simulink model "untitled"  (R2015b)
settings: Solver=VariableStepAuto  StartTime=0.0  StopTime=10.0  RelTol=1e-3
libraries: fl_lib x5, simulink_extras x2, simrfV2junction1 x2, commsynccomp2 x1
settings Model: Creator=dimple  LastModifiedBy=dimple

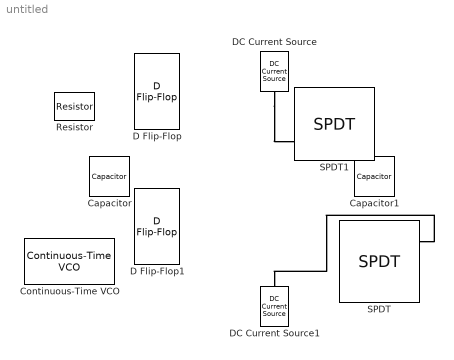
== system untitled ==
  Capacitor : fl_lib/Electrical/Electrical Elements/Capacitor  c=1e-6 F  r=1e-6 Ohm  g=0 1/Ohm  i_specify=off  i_priority=None  i=0 A  v_specify=off  v_priority=None  v=0 V  vc_specify=off  vc_priority=None  vc=0 V
  Capacitor1 : fl_lib/Electrical/Electrical Elements/Capacitor  c=1e-6 F  r=1e-6 Ohm  g=0 1/Ohm  i_specify=off  i_priority=None  i=0 A  v_specify=off  v_priority=None  v=0 V  vc_specify=off  vc_priority=None  vc=0 V
  Continuous-Time VCO : commsynccomp2/Continuous-Time VCO  Ac=1  Fc=10  Kc=1  Ph=0
  D Flip-Flop : simulink_extras/Flip Flops/D Flip-Flop
  D Flip-Flop1 : simulink_extras/Flip Flops/D Flip-Flop
  DC Current Source : fl_lib/Electrical/Electrical Sources/DC Current Source  i0=1 A
  DC Current Source1 : fl_lib/Electrical/Electrical Sources/DC Current Source  i0=1 A
  Resistor : fl_lib/Electrical/Electrical Elements/Resistor  R=1 Ohm  i_specify=off  i_priority=None  i=0 A  v_specify=off  v_priority=None  v=0 V
  SPDT : simrfV2junction1/SPDT  classname=spdt  SwitchType=switchSPDT  Vthres=0 V  CharType=Resistance  Ron=10 Ohm  Roff=1e6 Ohm  Iloss=1  Iiso=70  LoadType=Reflective  Z0=50 Ohm  InternalGrounding=on
  SPDT1 : simrfV2junction1/SPDT  classname=spdt  SwitchType=switchSPDT  Vthres=0 V  CharType=Resistance  Ron=10 Ohm  Roff=1e6 Ohm  Iloss=1  Iiso=70  LoadType=Reflective  Z0=50 Ohm  InternalGrounding=on
  connections:
  DC Current Source/LConn1 -- SPDT1/LConn1
  SPDT/RConn1 -- DC Current Source1/RConn1
